simulink model "model"  (R2021b)
settings: Solver=VariableStepAuto  StartTime=0.0  StopTime=10.0  RelTol=1e-3
values from neighbouring files (symbols this model uses):
  G = 9.81    [edda.m]
  O1 = 3.1    [edda.m]
  O2 = 9.5    [edda.m]
  O3 = 0.24    [edda.m]
  O4 = 0.77    [edda.m]
settings Model: Creator=mbober  LastModifiedBy=mbober
settings SolverCC: AlgebraicLoopSolver=TrustRegion
settings DebuggingCC: SFMachineParentedDataDiag=warning

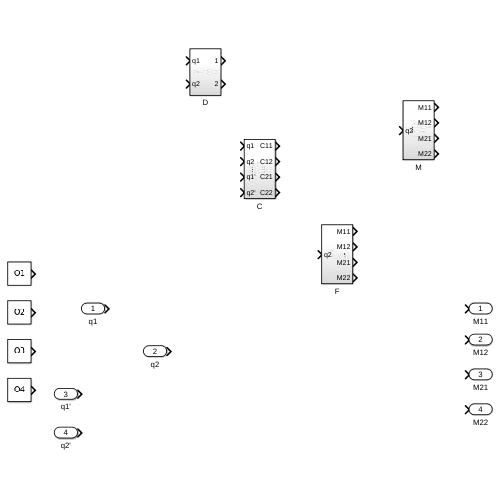
[thumbnail: Simulink's stored preview of the top-level diagram]
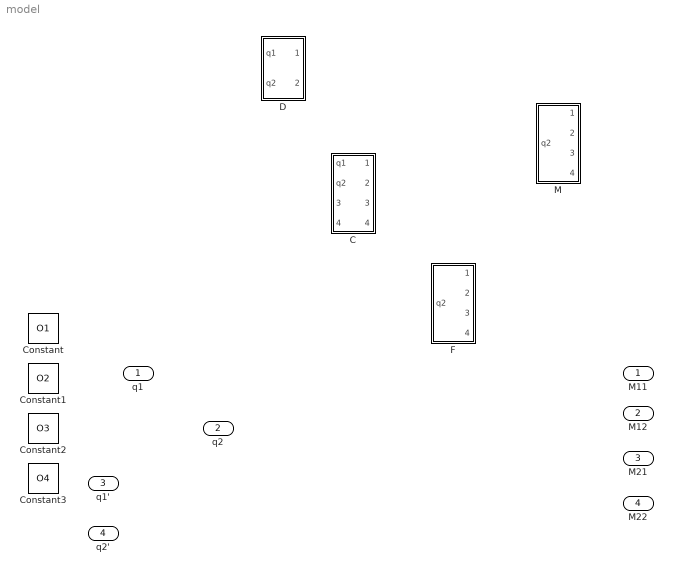
== system model ==
  q1 : Inport
  q2 : Inport  Port=2
  q1' : Inport  Port=3
  q2' : Inport  Port=4
  C : Subsystem
  Constant : Constant  Value=O1
  Constant1 : Constant  Value=O2
  Constant2 : Constant  Value=O3
  Constant3 : Constant  Value=O4
  D : Subsystem
  F : Subsystem
  M : Subsystem
  M11 : Outport
  M12 : Outport  Port=2
  M21 : Outport  Port=3
  M22 : Outport  Port=4

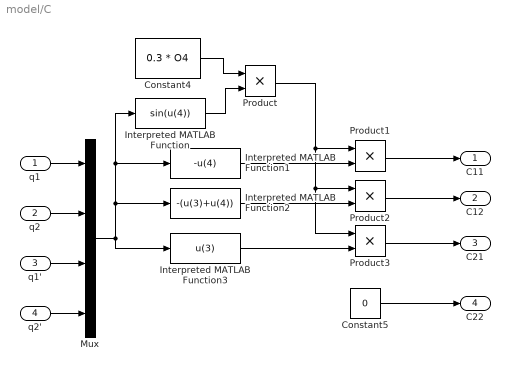
== system model/C ==
  q1 : Inport
  q2 : Inport  Port=2
  q1' : Inport  Port=3
  q2' : Inport  Port=4
  Constant4 : Constant  Value=0.3 * O4
  Constant5 : Constant  Value=0
  Interpreted MATLAB Function : MATLABFcn  MATLABFcn=sin(u(4))
  Interpreted MATLAB Function1 : MATLABFcn  MATLABFcn=-u(4)
  Interpreted MATLAB Function2 : MATLABFcn  MATLABFcn=-(u(3)+u(4))
  Interpreted MATLAB Function3 : MATLABFcn  MATLABFcn=u(3)
  Mux : Mux
  Product{,1..3} (4 alike) : Product
  C11 : Outport
  C12 : Outport  Port=2
  C21 : Outport  Port=3
  C22 : Outport  Port=4
  wires:
  Product3/1 -> C21/1
  Interpreted MATLAB Function1/1 -> Product1/2
  q2'/1 -> Mux/4
  Interpreted MATLAB Function2/1 -> Product2/2
  q2/1 -> Mux/2
  Constant4/1 -> Product/1
  Interpreted MATLAB Function/1 -> Product/2
  Product1/1 -> C11/1
  Interpreted MATLAB Function3/1 -> Product3/2
  q1'/1 -> Mux/3
  Mux/1 -> Interpreted MATLAB Function3/1, Interpreted MATLAB Function2/1, Interpreted MATLAB Function/1, Interpreted MATLAB Function1/1
  q1/1 -> Mux/1
  Constant5/1 -> C22/1
  Product/1 -> Product3/1, Product2/1, Product1/1
  Product2/1 -> C12/1

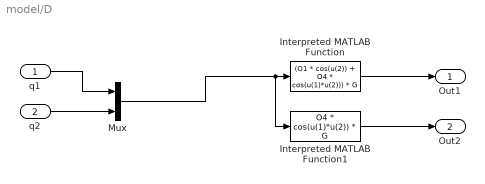
== system model/D ==
  q1 : Inport
  q2 : Inport  Port=2
  Interpreted MATLAB Function : MATLABFcn  MATLABFcn=(O1 * cos(u(2)) + O4 * cos(u(1)*u(2))) * G
  Interpreted MATLAB Function1 : MATLABFcn  MATLABFcn=O4 * cos(u(1)*u(2)) * G
  Mux : Mux  Inputs=2
  Out1 : Outport
  Out2 : Outport  Port=2
  wires:
  Interpreted MATLAB Function/1 -> Out1/1
  Interpreted MATLAB Function1/1 -> Out2/1
  Mux/1 -> Interpreted MATLAB Function1/1, Interpreted MATLAB Function/1
  q1/1 -> Mux/1
  q2/1 -> Mux/2

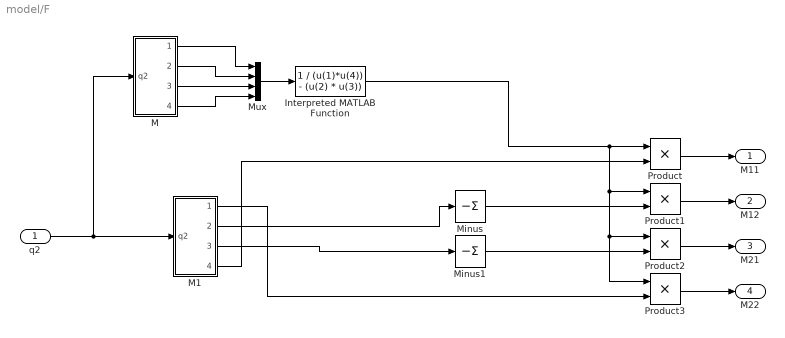
== system model/F ==
  q2 : Inport
  Interpreted MATLAB Function : MATLABFcn  MATLABFcn=1 / (u(1)*u(4)) - (u(2) * u(3))
  M : Subsystem
  M1 : Subsystem
  Minus : Sum  Inputs=-
  Minus1 : Sum  Inputs=-
  Mux : Mux
  Product{,1..3} (4 alike) : Product
  M11 : Outport
  M12 : Outport  Port=2
  M21 : Outport  Port=3
  M22 : Outport  Port=4
  wires:
  q2/1 -> M/1(q2), M1/1(q2)
  M1/2(M12) -> Minus/1
  M1/3(M21) -> Minus1/1
  Mux/1 -> Interpreted MATLAB Function/1
  M/2(M12) -> Mux/2
  M/1(M11) -> Mux/1
  M/3(M21) -> Mux/3
  M/4(M22) -> Mux/4
  Product/1 -> M11/1
  Product1/1 -> M12/1
  Product2/1 -> M21/1
  Product3/1 -> M22/1
  Interpreted MATLAB Function/1 -> Product3/1, Product2/1, Product1/1, Product/1
  M1/1(M11) -> Product3/2
  M1/4(M22) -> Product/2
  Minus/1 -> Product1/2
  Minus1/1 -> Product2/2

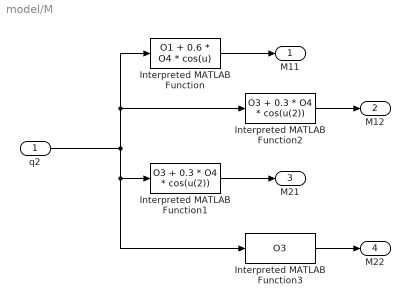
== system model/M ==
  q2 : Inport
  Interpreted MATLAB Function : MATLABFcn  MATLABFcn=O1 + 0.6 * O4 * cos(u)
  Interpreted MATLAB Function1 : MATLABFcn  MATLABFcn=O3 + 0.3 * O4 * cos(u(2))
  Interpreted MATLAB Function2 : MATLABFcn  MATLABFcn=O3 + 0.3 * O4 * cos(u(2))
  Interpreted MATLAB Function3 : MATLABFcn  MATLABFcn=O3
  M11 : Outport
  M12 : Outport  Port=2
  M21 : Outport  Port=3
  M22 : Outport  Port=4
  wires:
  Interpreted MATLAB Function3/1 -> M22/1
  Interpreted MATLAB Function/1 -> M11/1
  Interpreted MATLAB Function2/1 -> M12/1
  q2/1 -> Interpreted MATLAB Function/1, Interpreted MATLAB Function2/1, Interpreted MATLAB Function3/1, Interpreted MATLAB Function1/1
  Interpreted MATLAB Function1/1 -> M21/1

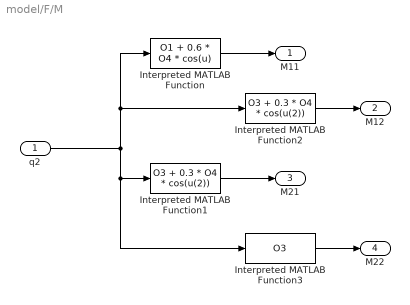
== system model/F/M ==
  q2 : Inport
  Interpreted MATLAB Function : MATLABFcn  MATLABFcn=O1 + 0.6 * O4 * cos(u)
  Interpreted MATLAB Function1 : MATLABFcn  MATLABFcn=O3 + 0.3 * O4 * cos(u(2))
  Interpreted MATLAB Function2 : MATLABFcn  MATLABFcn=O3 + 0.3 * O4 * cos(u(2))
  Interpreted MATLAB Function3 : MATLABFcn  MATLABFcn=O3
  M11 : Outport
  M12 : Outport  Port=2
  M21 : Outport  Port=3
  M22 : Outport  Port=4
  wires:
  Interpreted MATLAB Function3/1 -> M22/1
  Interpreted MATLAB Function/1 -> M11/1
  Interpreted MATLAB Function2/1 -> M12/1
  q2/1 -> Interpreted MATLAB Function/1, Interpreted MATLAB Function2/1, Interpreted MATLAB Function3/1, Interpreted MATLAB Function1/1
  Interpreted MATLAB Function1/1 -> M21/1

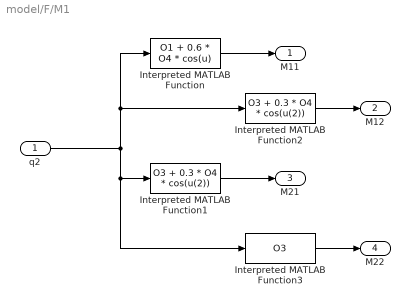
== system model/F/M1 ==
  q2 : Inport
  Interpreted MATLAB Function : MATLABFcn  MATLABFcn=O1 + 0.6 * O4 * cos(u)
  Interpreted MATLAB Function1 : MATLABFcn  MATLABFcn=O3 + 0.3 * O4 * cos(u(2))
  Interpreted MATLAB Function2 : MATLABFcn  MATLABFcn=O3 + 0.3 * O4 * cos(u(2))
  Interpreted MATLAB Function3 : MATLABFcn  MATLABFcn=O3
  M11 : Outport
  M12 : Outport  Port=2
  M21 : Outport  Port=3
  M22 : Outport  Port=4
  wires:
  Interpreted MATLAB Function3/1 -> M22/1
  Interpreted MATLAB Function/1 -> M11/1
  Interpreted MATLAB Function2/1 -> M12/1
  q2/1 -> Interpreted MATLAB Function/1, Interpreted MATLAB Function2/1, Interpreted MATLAB Function3/1, Interpreted MATLAB Function1/1
  Interpreted MATLAB Function1/1 -> M21/1
